simulink model "MotorCtrl_DTC_Math"  (R2023b)
settings: Solver=FixedStepDiscrete  StartTime=0.0  StopTime=5  FixedStep=MC_Sim_BaseStep  RelTol=1e-3  EnableMultiTasking=on
values from neighbouring files (symbols this model uses):
  MC_ADC_BitNum = 0.0    [MotorControlDataDictionary_Math.sldd]
  MC_ADC_Offset = 0.0    [MotorControlDataDictionary_Math.sldd]
  MC_ADC_VRef = 1.0    [MotorControlDataDictionary_Math.sldd]
  MC_Const_DutyL = 0.2    [MotorControlDataDictionary_Math.sldd]
  MC_Const_DutyS = 0.8    [MotorControlDataDictionary_Math.sldd]
  MC_CSA_Gain = 1.0    [MotorControlDataDictionary_Math.sldd]
  MC_Input_Vdc = 13.5    [MotorControlDataDictionary_Math.sldd]
  MC_MOS_DeadTime = 1.0E-6    [MotorControlDataDictionary_Math.sldd]
  MC_Motor_Mechinal_Damp = 1.0E-5    [MotorControlDataDictionary_Math.sldd]
  MC_Motor_Mechinal_Fric = 0.0    [MotorControlDataDictionary_Math.sldd]
  MC_Motor_Mechinal_Inertia = 0.0103    [MotorControlDataDictionary_Math.sldd]
  MC_Motor_Phi = 0.0059190254913385806    [MotorControlDataDictionary_Math.sldd]
  MC_Motor_Rotor_Pn = 4.0    [MotorControlDataDictionary_Math.sldd]
  MC_Motor_Stator_Ld = 5.6345E-5    [MotorControlDataDictionary_Math.sldd]
  MC_Motor_Stator_Lq = 5.6345E-5    [MotorControlDataDictionary_Math.sldd]
  MC_Motor_Stator_Rs = 0.0286    [MotorControlDataDictionary_Math.sldd]
  MC_Param_CurrentPI_Ki = 0.0071879639914134473    [MotorControlDataDictionary_Math.sldd]
  MC_Param_CurrentPI_Kp = 0.283220860906427    [MotorControlDataDictionary_Math.sldd]
  MC_Param_CurrentPI_UdInteMax = 7.794228634059948    [MotorControlDataDictionary_Math.sldd]
  MC_Param_CurrentPI_UdInteMin = -7.794228634059948    [MotorControlDataDictionary_Math.sldd]
  MC_Param_CurrentPI_UdMax = 7.794228634059948    [MotorControlDataDictionary_Math.sldd]
  MC_Param_CurrentPI_UdMin = -7.794228634059948    [MotorControlDataDictionary_Math.sldd]
  MC_Param_CurrentPI_UqInteMax = 7.794228634059948    [MotorControlDataDictionary_Math.sldd]
  MC_Param_CurrentPI_UqInteMin = -7.794228634059948    [MotorControlDataDictionary_Math.sldd]
  MC_Param_CurrentPI_UqMax = 7.794228634059948    [MotorControlDataDictionary_Math.sldd]
  MC_Param_CurrentPI_UqMin = -7.794228634059948    [MotorControlDataDictionary_Math.sldd]
  MC_Param_Flux_Gamma = 750000.0    [MotorControlDataDictionary_Math.sldd]
  MC_Param_Flux_Lalpha = 5.6345E-5    [MotorControlDataDictionary_Math.sldd]
  MC_Param_Flux_Lbeta = 5.6345E-5    [MotorControlDataDictionary_Math.sldd]
  MC_Param_Flux_Ralpha = 0.0286    [MotorControlDataDictionary_Math.sldd]
  MC_Param_Flux_Rbeta = 0.0286    [MotorControlDataDictionary_Math.sldd]
  MC_Param_Luen_BEMFalpha = -17747.803709290976    [MotorControlDataDictionary_Math.sldd]
  MC_Param_Luen_BEMFbeta = -17747.803709290976    [MotorControlDataDictionary_Math.sldd]
  MC_Param_Luen_BEMFErr = -8.0    [MotorControlDataDictionary_Math.sldd]
  MC_Param_Luen_Currentalpha = -507.58718608572195    [MotorControlDataDictionary_Math.sldd]
  MC_Param_Luen_Currentbeta = -507.58718608572195    [MotorControlDataDictionary_Math.sldd]
  MC_Param_Luen_CurrentErr = -8.0    [MotorControlDataDictionary_Math.sldd]
  MC_Param_Luen_PLL_Ki = 2.3480975196640594    [MotorControlDataDictionary_Math.sldd]
  MC_Param_Luen_PLL_Kp = 153.24842212633141    [MotorControlDataDictionary_Math.sldd]
  MC_Param_Luen_Voltagealpha = 17747.803709290976    [MotorControlDataDictionary_Math.sldd]
  MC_Param_Luen_Voltagebeta = 17747.803709290976    [MotorControlDataDictionary_Math.sldd]
  MC_Param_PhasetoReal = 500.0    [MotorControlDataDictionary_Math.sldd]
  MC_Param_SMO_CoffA = 0.97462064069571386    [MotorControlDataDictionary_Math.sldd]
  MC_Param_SMO_CoffB = 0.88739018546454884    [MotorControlDataDictionary_Math.sldd]
  MC_Param_SpeedCtrl_IdMax = 60.0    [MotorControlDataDictionary_Math.sldd]
  MC_Param_SpeedCtrl_IdMin = -60.0    [MotorControlDataDictionary_Math.sldd]
  MC_Param_SpeedCtrl_IqMax = 60.0    [MotorControlDataDictionary_Math.sldd]
  MC_Param_SpeedCtrl_IqMin = -60.0    [MotorControlDataDictionary_Math.sldd]
  MC_Param_SpeedPI_Ki = 0.57248683633241571    [MotorControlDataDictionary_Math.sldd]
  MC_Param_SpeedPI_Kp = 9.1114109857344836    [MotorControlDataDictionary_Math.sldd]
  MC_Param_SpeedtoTheta = 5.0E-5    [MotorControlDataDictionary_Math.sldd]
  MC_Param_SVPWM_DutyMax = 0.98    [MotorControlDataDictionary_Math.sldd]
  MC_Param_SVPWM_DutyMin = 0.02    [MotorControlDataDictionary_Math.sldd]
  MC_Param_SVPWM_SampleOffset1 = 0.02    [MotorControlDataDictionary_Math.sldd]
  MC_Param_SVPWM_SampleOffset2 = 0.015    [MotorControlDataDictionary_Math.sldd]
  MC_Param_SVPWM_SampleValid = 0.011999999999999999    [MotorControlDataDictionary_Math.sldd]
  MC_Sample_CurrentNoise = 1.0E-15    [MotorControlDataDictionary_Math.sldd]
  MC_Sample_Rs = 0.002    [MotorControlDataDictionary_Math.sldd]
  MC_Sample_VbusNoise = 1.0E-15    [MotorControlDataDictionary_Math.sldd]
  MC_Sim_BaseStep = 5.0E-8    [MotorControlDataDictionary_Math.sldd]
  MC_Sim_HFTStep = 5.0E-5    [MotorControlDataDictionary_Math.sldd]
  MC_Sim_MFTStep = 0.002    [MotorControlDataDictionary_Math.sldd]
libraries: simulink x29, spsVoltageMeasurementLib x2, spsDCVoltageSourceLib x1, spsGroundLib x1, spsPermanentMagnetSynchronousMachineLib x1, spsSeriesRLCBranchLib x1, spsThreePhaseVIMeasurementLib x1, spsUniversalBridgeLib x1, sps_lib x1
(part 4 of 5)

== system MotorCtrl_DTC_Math/HFTask/smo/getSpeedandTheta ==
  note: 日志：
      | 2025.03.19：反电势正负号识别错误，改正后可以使用
  Ealpha : Inport
  Ebeta : Inport  Port=2
  Add : Sum
  Add1 : Sum
  Add2 : Sum
  Constant : Constant  Value=2*pi  OutDataTypeStr=single
  Delay One Step : Delay  DelayLength=1
  Delay One Step2 : Delay  DelayLength=1
  Gain : Gain  Gain=-1
  Gain1 : Gain  Gain=2*sqrt(2)/2*100
  Gain2 : Gain  Gain=100^2*MC_Sim_HFTStep
  Gain3 : Gain  Gain=MC_Param_SpeedtoTheta
  Gain5 : Gain  Gain=30/(pi*MC_Motor_Rotor_Pn)  OutDataTypeStr=single  RndMeth=Simplest
  Mod : Math  Operator=mod
  Product : Product
  Product1 : Product
  Sin : Trigonometry  OutputSignalType=real
  Sin1 : Trigonometry  Operator=cos  OutputSignalType=real
  Subtract : Sum  Inputs=+-
  Speed : Outport
  Theta : Outport  Port=2
  wires:
  Sin1/1 -> Product/2
  Sin/1 -> Product1/2
  Gain2/1 -> Add/1
  Add/1 -> Delay One Step/1, Add1/2
  Delay One Step/1 -> Add/2
  Gain1/1 -> Add1/1
  Subtract/1 -> Gain2/1, Gain1/1  "SMOErr"
  Gain3/1 -> Add2/1
  Add2/1 -> Mod/1
  Constant/1 -> Mod/2
  Delay One Step2/1 -> Add2/2, [Theta_Last]
  Mod/1 -> Theta/1, Delay One Step2/1  "ThetaSMO"
  Add1/1 -> Gain5/1, Gain3/1  "SpeedSmo"
  [Theta_Last] -> Sin1/1, Sin/1
  Gain/1 -> Product1/1
  Ebeta/1 -> Gain/1
  Ealpha/1 -> Product/1
  Product/1 -> Subtract/1  "SMOSin"
  Product1/1 -> Subtract/2  "SMOCos"
  Gain5/1 -> Speed/1  "SpeedSMO_RPM"

== system MotorCtrl_DTC_Math/HFTask/svpwm/getVoltageExchange ==
  Valpha : Inport
  Vbeta : Inport  Port=2
  Vdc : Inport  Port=3
  Add : Sum
  Add1 : Sum
  Divide : Product  Inputs=*/
  Divide1 : Product  Inputs=*/
  Gain : Gain  Gain=-1/2
  Gain1 : Gain  Gain=sqrt(3)/2
  Gain2 : Gain  Gain=-1
  Relational Operator : RelationalOperator  OutDataTypeStr=boolean  RndMeth=Simplest  InputSameDT=off
  Relational Operator1 : RelationalOperator  OutDataTypeStr=boolean  RndMeth=Simplest  InputSameDT=off
  Relational Operator2 : RelationalOperator  Operator=<=  OutDataTypeStr=boolean  RndMeth=Simplest  InputSameDT=off
  Relational Operator3 : RelationalOperator  Operator=<=  OutDataTypeStr=boolean  RndMeth=Simplest  InputSameDT=off
  Signal Copy : SignalConversion  OverrideOpt=off
  Subtract : Sum  Inputs=+-
  Switch{,1..3} (4 alike) : Switch  Criteria=u2 > Threshold  SaturateOnIntegerOverflow=off  InputSameDT=off
  getSectorN : Subsystem  Commented=on
  Va : Outport
  Vb : Outport  Port=2
  Vc : Outport  Port=3
  Vmed : Outport  Port=4
  wires:
  Valpha/1 -> Divide/1
  Vbeta/1 -> Divide1/1
  Vdc/1 -> Divide/2, Divide1/2
  Subtract/1 -> Relational Operator3/2, Switch3/3, Relational Operator1/2, Switch1/3, Vc/1  "Vc"
  Add/1 -> Switch2/3, Relational Operator2/2, Switch/3, Relational Operator/2, Vb/1  "Vb"
  Gain1/1 -> Subtract/2, Add/2
  Gain/1 -> Add/1, Subtract/1
  Divide1/1 -> Gain1/1
  Divide/1 -> Gain/1, Signal Copy/1
  Signal Copy/1 -> Switch2/1, Relational Operator2/1, Switch/1, Relational Operator/1, Va/1  "Va"
  Switch1/1 -> Add1/1  "Vmax"
  Relational Operator1/1 -> Switch1/2
  Switch/1 -> Relational Operator1/1, Switch1/1
  Relational Operator/1 -> Switch/2
  Switch3/1 -> Add1/2  "Vmin"
  Relational Operator3/1 -> Switch3/2
  Switch2/1 -> Switch3/1, Relational Operator3/1
  Relational Operator2/1 -> Switch2/2
  Add1/1 -> Gain2/1
  Gain2/1 -> Vmed/1  "Vmed"

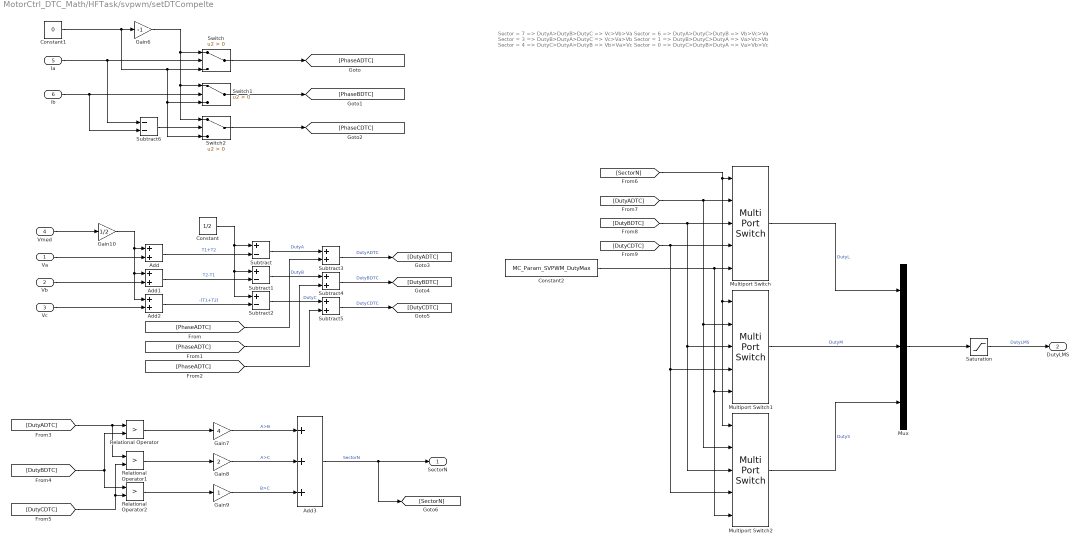
== system MotorCtrl_DTC_Math/HFTask/svpwm/setDTCompelte ==
  note: Sector = 7 => DutyA>DutyB>DutyC => Vc>Vb>Va
      | Sector = 6 => DutyA>DutyC>DutyB => Vb>Vc>Va
      | Sector = 3 => DutyB>DutyA>DutyC => Vc>Va>Vb
      | Sector = 1 => DutyB>DutyC>DutyA => Va>Vc>Vb
      | Sector = 4 => DutyC>DutyA>DutyB => Vb>Va>Vc
      | Sector = 0 => DutyC>DutyB>DutyA => Va>Vb>Vc
  Va : Inport
  Vb : Inport  Port=2
  Vc : Inport  Port=3
  Vmed : Inport  Port=4
  Ia : Inport  Port=5
  ib : Inport  Port=6
  Add : Sum
  Add1 : Sum
  Add2 : Sum
  Add3 : Sum  Inputs=+++
  Constant : Constant  Value=1/2  OutDataTypeStr=single  SampleTime=MC_Sim_HFTStep
  Constant1 : Constant  Value=0  OutDataTypeStr=single
  Constant2 : Constant  Value=MC_Param_SVPWM_DutyMax  OutDataTypeStr=single
  Gain10 : Gain  Gain=1/2
  Gain6 : Gain  Gain=-1
  Gain7 : Gain  Gain=4  OutDataTypeStr=single  RndMeth=Simplest
  Gain8 : Gain  Gain=2  OutDataTypeStr=single  RndMeth=Simplest
  Gain9 : Gain  OutDataTypeStr=single  RndMeth=Simplest
  Multiport Switch : MultiPortSwitch  DataPortOrder=Specify indices  DataPortIndices={[6,7],[1,3],[0,4]}  DataPortForDefault=Additional data port  SaturateOnIntegerOverflow=off  InputSameDT=off
  Multiport Switch1 : MultiPortSwitch  DataPortOrder=Specify indices  DataPortIndices={[4,3],[7,0],[6,1]}  DataPortForDefault=Additional data port  SaturateOnIntegerOverflow=off  InputSameDT=off
  Multiport Switch2 : MultiPortSwitch  DataPortOrder=Specify indices  DataPortIndices={[0,1],[4,6],[3,7]}  DataPortForDefault=Additional data port  SaturateOnIntegerOverflow=off  InputSameDT=off
  Mux : Mux  Inputs=3
  Relational Operator : RelationalOperator  Operator=>  OutDataTypeStr=boolean  RndMeth=Simplest  InputSameDT=off
  Relational Operator1 : RelationalOperator  Operator=>  OutDataTypeStr=boolean  RndMeth=Simplest  InputSameDT=off
  Relational Operator2 : RelationalOperator  Operator=>  OutDataTypeStr=boolean  RndMeth=Simplest  InputSameDT=off
  Saturation : Saturate  UpperLimit=MC_Param_SVPWM_DutyMax-(MC_MOS_DeadTime/MC_Sim_HFTStep)  LowerLimit=MC_Param_SVPWM_DutyMin+(MC_MOS_DeadTime/MC_Sim_HFTStep)
      settings: AttributesFormatString=|
      | OutputMax = %<UpperLimit>
      | OutputMin = %<LowerLimit>
  Subtract : Sum  Inputs=+-
  Subtract1 : Sum  Inputs=+-
  Subtract2 : Sum  Inputs=+-
  Subtract3 : Sum
  Subtract4 : Sum
  Subtract5 : Sum
  Subtract6 : Sum  Inputs=--
  Switch : Switch  Criteria=u2 > Threshold  SaturateOnIntegerOverflow=off  InputSameDT=off
  Switch1 : Switch  Criteria=u2 > Threshold  SaturateOnIntegerOverflow=off  InputSameDT=off
  Switch2 : Switch  Criteria=u2 > Threshold  SaturateOnIntegerOverflow=off  InputSameDT=off
  SectorN : Outport
  DutyLMS : Outport  Port=2
  wires:
  Va/1 -> Add/2
  Vmed/1 -> Gain10/1
  Vb/1 -> Add1/2
  Vc/1 -> Add2/2
  Add/1 -> Subtract/2  "T1+T2"
  Add2/1 -> Subtract2/2  "-(T1+T2)"
  Add1/1 -> Subtract1/2  "T2-T1"
  Constant/1 -> Subtract2/1, Subtract1/1, Subtract/1
  Subtract/1 -> Subtract3/1  "DutyA"
  Subtract1/1 -> Subtract4/1  "DutyB"
  Subtract2/1 -> Subtract5/1  "DutyC"
  Ia/1 -> Subtract6/1, Switch/2
  Gain6/1 -> Switch2/1, Switch1/1, Switch/1
  ib/1 -> Subtract6/2, Switch1/2
  Subtract6/1 -> Switch2/2
  Constant1/1 -> Switch2/3, Switch1/3, Switch/3, Gain6/1
  Switch/1 -> [PhaseADTC]
  Switch1/1 -> [PhaseBDTC]
  Switch2/1 -> [PhaseCDTC]
  [PhaseADTC] -> Subtract3/2
  [PhaseADTC] -> Subtract4/2
  [PhaseADTC] -> Subtract5/2
  [DutyBDTC] -> Relational Operator/2, Relational Operator2/1
  [DutyADTC] -> Relational Operator1/1, Relational Operator/1
  [DutyCDTC] -> Relational Operator2/2, Relational Operator1/2
  Relational Operator/1 -> Gain7/1
  Relational Operator1/1 -> Gain8/1
  Relational Operator2/1 -> Gain9/1
  Gain8/1 -> Add3/2  "A>C"
  Gain9/1 -> Add3/3  "B>C"
  Gain7/1 -> Add3/1  "A>B"
  Add3/1 -> [SectorN], SectorN/1  "SectorN"
  Gain10/1 -> Add2/1, Add1/1, Add/1
  Subtract3/1 -> [DutyADTC]  "DutyADTC"
  Subtract4/1 -> [DutyBDTC]  "DutyBDTC"
  Subtract5/1 -> [DutyCDTC]  "DutyCDTC"
  [SectorN] -> Multiport Switch2/1, Multiport Switch1/1, Multiport Switch/1
  Multiport Switch/1 -> Mux/1  "DutyL"
  Constant2/1 -> Multiport Switch2/5, Multiport Switch1/5, Multiport Switch/5
  Multiport Switch1/1 -> Mux/2  "DutyM"
  Multiport Switch2/1 -> Mux/3  "DutyS"
  Mux/1 -> Saturation/1
  Saturation/1 -> DutyLMS/1  "DutyLMS"
  [DutyADTC] -> Multiport Switch2/2, Multiport Switch1/2, Multiport Switch/2
  [DutyCDTC] -> Multiport Switch2/4, Multiport Switch1/4, Multiport Switch/4
  [DutyBDTC] -> Multiport Switch2/3, Multiport Switch1/3, Multiport Switch/3

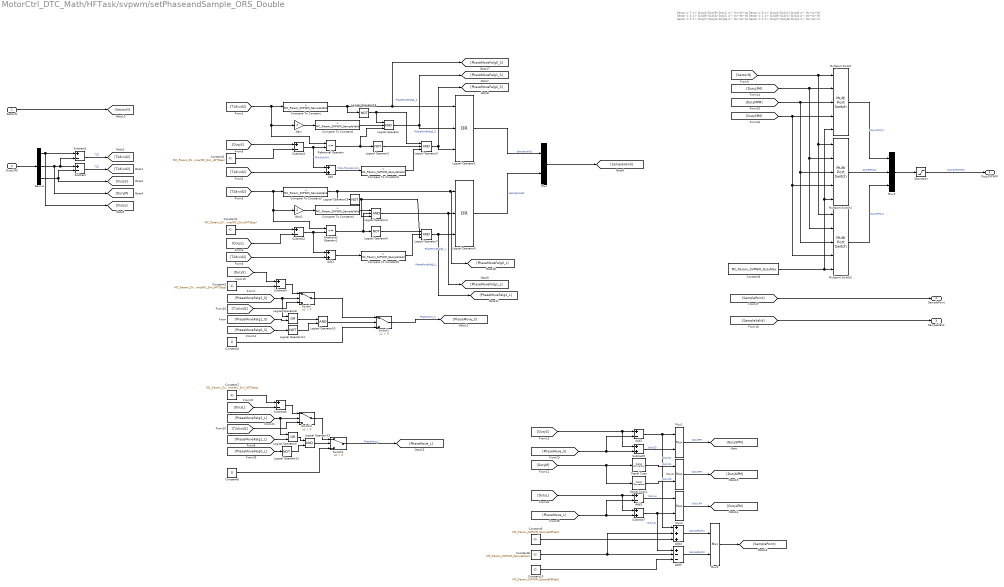
== system MotorCtrl_DTC_Math/HFTask/svpwm/setPhaseandSample_ORS_Double ==
  note: Sector = 7 => DutyA>DutyB>DutyC => Vc>Vb>Va
      | Sector = 6 => DutyA>DutyC>DutyB => Vb>Vc>Va
      | Sector = 3 => DutyB>DutyA>DutyC => Vc>Va>Vb
      | Sector = 1 => DutyB>DutyC>DutyA => Va>Vc>Vb
      | Sector = 4 => DutyC>DutyA>DutyB => Vb>Va>Vc
      | Sector = 0 => DutyC>DutyB>DutyA => Va>Vb>Vc
  SectorN : Inport
  DutyLMS : Inport  Port=2
  Add : Sum
  Add1 : Sum
  Add2 : Sum  Inputs=+-
  Add3 : Sum  Inputs=+-
  Add4 : Sum  Inputs=+++
  Add5 : Sum  Inputs=+--
  Compare To Constant{,1..5} (6 alike) : simulink/Logic and Bit Operations/Compare To Constant  relop=>  const=MC_Param_SVPWM_SampleValid  OutDataTypeStr=boolean
  Constant1 : Constant  Value=MC_Param_SVPWM_DutyMax-(MC_MOS_DeadTime/MC_Sim_HFTStep)  OutDataTypeStr=single
  Constant10 : Constant  Value=MC_Param_SVPWM_SampleOffset2  OutDataTypeStr=single
  Constant2 : Constant  Value=MC_Param_SVPWM_DutyMin+(MC_MOS_DeadTime/MC_Sim_HFTStep)  OutDataTypeStr=single
  Constant3 : Constant  Value=MC_Param_SVPWM_DutyMin+(MC_MOS_DeadTime/MC_Sim_HFTStep)  OutDataTypeStr=single
  Constant4 : Constant  Value=0  OutDataTypeStr=single
  Constant5 : Constant  Value=MC_Param_SVPWM_DutyMax  OutDataTypeStr=single
  Constant6 : Constant  Value=0  OutDataTypeStr=single
  Constant7 : Constant  Value=MC_Param_SVPWM_DutyMax-(MC_MOS_DeadTime/MC_Sim_HFTStep)  OutDataTypeStr=single
  Constant8 : Constant  Value=MC_Param_SVPWM_SampleValid  OutDataTypeStr=single
  Constant9 : Constant  Value=MC_Param_SVPWM_SampleOffset1  OutDataTypeStr=single
  Demux : Demux  Outputs=3
  Gain : Gain  Gain=2
  Gain1 : Gain  Gain=2
  Logical Operator{,3..4,7} (4 alike) : Logic  Inputs=3  AllPortsSameDT=off  OutDataTypeStr=boolean
  Logical Operator1 : Logic  Operator=OR  Inputs=3  AllPortsSameDT=off  OutDataTypeStr=boolean
  Logical Operator10 : Logic  AllPortsSameDT=off  OutDataTypeStr=boolean
  Logical Operator{2,6,11..12,14..15} (6 alike) : Logic  Operator=NOT  AllPortsSameDT=off  OutDataTypeStr=boolean
  Logical Operator13 : Logic  AllPortsSameDT=off  OutDataTypeStr=boolean
  Logical Operator5 : Logic  Operator=OR  Inputs=3  AllPortsSameDT=off  OutDataTypeStr=boolean
  Logical Operator8 : Logic  Operator=OR  AllPortsSameDT=off  OutDataTypeStr=boolean
  Logical Operator9 : Logic  Operator=OR  AllPortsSameDT=off  OutDataTypeStr=boolean
  Multiport Switch : MultiPortSwitch  DataPortOrder=Specify indices  DataPortIndices={[7,6],[3,4],[0,1]}  DataPortForDefault=Additional data port  SaturateOnIntegerOverflow=off  InputSameDT=off
  Multiport Switch1 : MultiPortSwitch  DataPortOrder=Specify indices  DataPortIndices={[3,1],[7,0],[6,4]}  DataPortForDefault=Additional data port  SaturateOnIntegerOverflow=off  InputSameDT=off
  Multiport Switch2 : MultiPortSwitch  DataPortOrder=Specify indices  DataPortIndices={[4,0],[6,1],[7,3]}  DataPortForDefault=Additional data port  SaturateOnIntegerOverflow=off  InputSameDT=off
  Mux{,1..4} (5 alike) : Mux  Inputs=2
  Mux5 : Mux  Inputs=3
  Relational Operator : RelationalOperator  Operator=<=  OutDataTypeStr=boolean  RndMeth=Simplest  InputSameDT=off
  Relational Operator1 : RelationalOperator  Operator=<=  OutDataTypeStr=boolean  RndMeth=Simplest  InputSameDT=off
  Saturation : Saturate  UpperLimit=MC_Param_SVPWM_DutyMax  LowerLimit=MC_Param_SVPWM_DutyMin
      settings: AttributesFormatString=|
      | OutputMax = %<UpperLimit>
      | OutputMin = %<LowerLimit>
  Signal Copy : SignalConversion  OverrideOpt=off
  Signal Copy1 : SignalConversion  OverrideOpt=off
  Subtract{,1..4,6} (6 alike) : Sum  Inputs=+-
  Subtract5 : Sum
  Subtract7 : Sum
  Switch{,1..3} (4 alike) : Switch  Criteria=u2 > Threshold  SaturateOnIntegerOverflow=off  InputSameDT=off
  DutySVPWM : Outport
  SamplePoint : Outport  Port=2
  SampleValid : Outport  Port=3
  wires:
  DutyLMS/1 -> Demux/1
  Subtract/1 -> [T1divid2]  "T1/2"
  Subtract1/1 -> [T2divid2]  "T2/2"
  SectorN/1 -> [SectorN]
  [SectorN] -> Multiport Switch2/1, Multiport Switch1/1, Multiport Switch/1
  [DutyLPM] -> Multiport Switch2/2, Multiport Switch1/2, Multiport Switch/2
  [DutyMPM] -> Multiport Switch2/3, Multiport Switch1/3, Multiport Switch/3
  [DutySPM] -> Multiport Switch1/4, Multiport Switch2/4, Multiport Switch/4
  Constant5/1 -> Multiport Switch1/5, Multiport Switch/5, Multiport Switch2/5
  Multiport Switch1/1 -> Mux5/2  "DutyBPM[2]"
  Multiport Switch2/1 -> Mux5/3  "DutyCPM[2]"
  Multiport Switch/1 -> Mux5/1  "DutyAPM[2]"
  [SamplePoint] -> SamplePoint/1
  [SampleValid] -> SampleValid/1
  Mux5/1 -> Saturation/1
  Saturation/1 -> DutySVPWM/1  "DutySVPWM[6]"
  [T1divid2] -> Relational Operator/1, Gain/1, Compare To Constant/1
  Gain/1 -> Compare To Constant1/1
  [DutyS] -> Subtract3/1
  Subtract3/1 -> Add/1, Relational Operator/2  "T0/4-DutyMin"
  Relational Operator/1 -> Logical Operator/3, Logical Operator2/1
  Logical Operator/1 -> Logical Operator1/2, [PhaseMoveFalg1_S]  "PhaseMoveFalg1_S"
  [T1divid2] -> Add/2
  Add/1 -> Compare To Constant2/1  "T1/2+T0/4-DutyMin"
  Compare To Constant/1 -> Logical Operator14/1, [PhaseMoveFalg0_S], Logical Operator1/1
  Logical Operator1/1 -> Mux/1  "SampleValid1"
  Logical Operator5/1 -> Mux/2  "SampleValid2"
  Compare To Constant3/1 -> Logical Operator15/1, [PhaseMoveFalg0_L], Logical Operator5/1
  Compare To Constant5/1 -> Logical Operator7/2
  Logical Operator6/1 -> Logical Operator7/1
  Logical Operator7/1 -> [PhaseMoveFalg2_L], Logical Operator5/3  "PhaseMoveFalg2_L"
  Add1/1 -> Compare To Constant5/1
  [T2divid2] -> Add1/2
  Logical Operator4/1 -> [PhaseMoveFalg1_L], Logical Operator5/2  "PhaseMoveFalg1_L"
  Relational Operator1/1 -> Logical Operator4/2, Logical Operator6/1
  Compare To Constant4/1 -> Logical Operator4/1
  Subtract2/1 -> Relational Operator1/2, Add1/1
  Constant1/1 -> Subtract2/1
  [DutyL] -> Subtract2/2
  Gain1/1 -> Compare To Constant4/1
  [T2divid2] -> Compare To Constant3/1, Gain1/1, Relational Operator1/1
  Constant2/1 -> Subtract3/2
  Mux/1 -> [SampleValid]
  Logical Operator3/1 -> Logical Operator1/3, [PhaseMoveFalg2_S]  "PhaseMoveFalg2_S"
  Constant3/1 -> Subtract4/2
  [DutyS] -> Subtract4/1
  [PhaseMoveFalg2_S] -> Logical Operator8/1, Switch/2
  Switch/1 -> Switch1/1
  Constant4/1 -> Switch1/3
  Switch1/1 -> [PhaseMove_S]  "PhaseMove_S"
  [T1divid2] -> Switch/3
  Subtract4/1 -> Switch/1
  Switch2/1 -> [PhaseMove_L]  "PhaseMove_L"
  Constant6/1 -> Switch2/3
  [T2divid2] -> Switch3/3
  Switch3/1 -> Switch2/1
  [DutyL] -> Subtract6/2
  Constant7/1 -> Subtract6/1
  Subtract6/1 -> Switch3/1
  Demux/1 -> [DutyL], Subtract1/1
  Demux/2 -> [DutyM], Subtract1/2, Subtract/1
  Demux/3 -> Subtract/2, [DutyS]
  [DutyS] -> Subtract5/1, Add2/1
  [PhaseMove_S] -> Add2/2, Subtract5/2
  Add2/1 -> Mux1/1, Add4/1  "DutySU"
  Subtract5/1 -> Mux1/2  "DutySD"
  Subtract7/1 -> Add5/1, Mux2/2  "DutyLD"
  Add3/1 -> Mux2/1  "DutyLU"
  [PhaseMove_L] -> Subtract7/2, Add3/2
  [DutyL] -> Add3/1, Subtract7/1
  [DutyM] -> Signal Copy1/1, Signal Copy/1
  Signal Copy1/1 -> Mux3/2  "DutyMD"
  Signal Copy/1 -> Mux3/1  "DutyMU"
  Mux1/1 -> [DutySPM]  "DutySPM"
  Mux2/1 -> [DutyLPM]  "DutyLPM"
  Mux3/1 -> [DutyMPM]  "DutyMPM"
  Constant8/1 -> Add4/2, Add5/2
  Add4/1 -> Mux4/1  "SamplePoint1"
  Add5/1 -> Mux4/2  "SamplePoint2"
  Mux4/1 -> [SamplePoint]
  Constant9/1 -> Add4/3
  Constant10/1 -> Add5/3
  [PhaseMoveFalg2_L] -> Logical Operator9/1, Switch3/2
  [PhaseMoveFalg1_L] -> Logical Operator9/2
  Logical Operator10/1 -> Switch1/2
  Logical Operator8/1 -> Logical Operator10/1
  [PhaseMoveFalg0_S] -> Logical Operator11/1
  Logical Operator11/1 -> Logical Operator10/2
  [PhaseMoveFalg1_S] -> Logical Operator8/2
  [PhaseMoveFalg0_L] -> Logical Operator12/1
  Logical Operator13/1 -> Switch2/2
  Logical Operator9/1 -> Logical Operator13/1
  Logical Operator12/1 -> Logical Operator13/2
  Compare To Constant1/1 -> Logical Operator/2
  Logical Operator14/1 -> Logical Operator3/1, Logical Operator/1
  Logical Operator2/1 -> Logical Operator3/2
  Compare To Constant2/1 -> Logical Operator3/3
  Logical Operator15/1 -> Logical Operator4/3, Logical Operator7/3

== system MotorCtrl_DTC_Math/Hardware_Math/PWMGenerate/DeadTimeGenerate ==
  FLag : Inport
  DutyABC : Inport  Port=2
  APhaseDeadTime : Subsystem
  BPhaseDeadTime : Subsystem
  CPhaseDeadTime : Subsystem
  Constant : Constant  Value=MC_MOS_DeadTime/MC_Sim_HFTStep  SampleTime=-1
  Demux : Demux  Outputs=6
  GateAH : Outport
  GateAL : Outport  Port=2
  GateBH : Outport  Port=3
  GateBL : Outport  Port=4
  GateCH : Outport  Port=5
  GateCL : Outport  Port=6
  wires:
  Demux/6 -> CPhaseDeadTime/3(CL)
  DutyABC/1 -> Demux/1
  CPhaseDeadTime/1(CDH) -> GateCH/1
  CPhaseDeadTime/2(CDL) -> GateCL/1
  BPhaseDeadTime/1(BDH) -> GateBH/1
  BPhaseDeadTime/2(BDL) -> GateBL/1
  APhaseDeadTime/2(ADL) -> GateAL/1
  FLag/1 -> CPhaseDeadTime/1(FLag), BPhaseDeadTime/1(FLag), APhaseDeadTime/1(FLag)
  Constant/1 -> APhaseDeadTime/4(DeadTime), BPhaseDeadTime/4(DeadTime), CPhaseDeadTime/4(DeadTime)
  APhaseDeadTime/1(ADH) -> GateAH/1
  Demux/5 -> BPhaseDeadTime/3(BL)
  Demux/4 -> APhaseDeadTime/3(AL)
  Demux/1 -> APhaseDeadTime/2(AH)
  Demux/2 -> BPhaseDeadTime/2(BH)
  Demux/3 -> CPhaseDeadTime/2(CH)

== system MotorCtrl_DTC_Math/Hardware_Math/currentSample/getCurrentSample_ORS_Double ==
  SampleTrigger : Inport
  Current : Inport  Port=2
  Demux : Demux  Outputs=2
  Mux : Mux  Inputs=2
  getCurrentSample1 : Subsystem  TreatAsAtomicUnit=on
  getCurrentSample2 : Subsystem  TreatAsAtomicUnit=on
  SampleCurrent : Outport
  wires:
  SampleTrigger/1 -> Demux/1
  Demux/1 -> getCurrentSample1/Trigger
  Demux/2 -> getCurrentSample2/Trigger
  Current/1 -> getCurrentSample2/1(Current), getCurrentSample1/1(Current)
  getCurrentSample1/1(SampleCurrentUp) -> Mux/1
  Mux/1 -> SampleCurrent/1
  getCurrentSample2/1(SampleCurrentDown) -> Mux/2

== system MotorCtrl_DTC_Math/Hardware_Math/currentSample/getCurrentSample_ORS_Single ==
  SampleTrigger : Inport
  Current : Inport  Port=2
  Demux : Demux  Outputs=2
  Mux : Mux  Inputs=2
  getCurrentSample1 : Subsystem  TreatAsAtomicUnit=on
  getCurrentSample2 : Subsystem  TreatAsAtomicUnit=on
  SampleCurrent : Outport
  wires:
  SampleTrigger/1 -> Demux/1
  Mux/1 -> SampleCurrent/1
  getCurrentSample1/1(SampleCurrentUp) -> Mux/1
  getCurrentSample2/1(SampleCurrentDown) -> Mux/2
  Demux/1 -> getCurrentSample1/Trigger
  Demux/2 -> getCurrentSample2/Trigger
  Current/1 -> getCurrentSample2/1(Current), getCurrentSample1/1(Current)

== system MotorCtrl_DTC_Math/Hardware_Math/currentSample/getCurrentSample_TRS(Three) ==
  SampleTrigger : Inport
  Current : Inport  Port=2
  Demux : Demux  Outputs=3
  Mux : Mux  Inputs=3
  getCurrentSampleA : Subsystem  TreatAsAtomicUnit=on
  getCurrentSampleB : Subsystem  TreatAsAtomicUnit=on
  getCurrentSampleC : Subsystem  TreatAsAtomicUnit=on
  SampleCurrent : Outport
  wires:
  getCurrentSampleA/1(SampleCurrentA) -> Mux/1
  getCurrentSampleB/1(SampleCurrentB) -> Mux/2
  Mux/1 -> SampleCurrent/1
  getCurrentSampleC/1(SampleCurrentC) -> Mux/3
  SampleTrigger/1 -> getCurrentSampleB/Trigger, getCurrentSampleC/Trigger, getCurrentSampleA/Trigger
  Current/1 -> Demux/1
  Demux/1 -> getCurrentSampleA/1(Current)
  Demux/2 -> getCurrentSampleB/1(Current)
  Demux/3 -> getCurrentSampleC/1(Current)

== system MotorCtrl_DTC_Math/Hardware_Math/currentSample/getCurrentSample_TRS(Two) ==
  SampleTrigger : Inport
  Current : Inport  Port=2
  Demux : Demux  Outputs=2
  Mux : Mux  Inputs=2
  getCurrentSample1 : Subsystem  TreatAsAtomicUnit=on
  getCurrentSample2 : Subsystem  TreatAsAtomicUnit=on
  SampleCurrent : Outport
  wires:
  Demux/1 -> getCurrentSample1/Trigger
  Current/1 -> getCurrentSample2/1(Current), getCurrentSample1/1(Current)
  Demux/2 -> getCurrentSample2/Trigger
  getCurrentSample1/1(SampleCurrentUp) -> Mux/1
  getCurrentSample2/1(SampleCurrentDown) -> Mux/2
  Mux/1 -> SampleCurrent/1
  SampleTrigger/1 -> Demux/1

== system MotorCtrl_DTC_Math/svpwm_OM/getVoltageExchange/getSectorN ==
  Valpha : Inport
  Vbeta : Inport  Port=2
  Add : Sum
  Add1 : Sum  Inputs=+++
  Constant : Constant
  Constant1 : Constant  Value=0
  Gain : Gain  Gain=sqrt(3)/2
  Gain1 : Gain  Gain=-1/2
  Gain2 : Gain
  Gain3 : Gain  Gain=2
  Gain4 : Gain  Gain=4
  Subtract : Sum  Inputs=-+
  Switch : Switch  Criteria=u2 > Threshold  SaturateOnIntegerOverflow=off  InputSameDT=off
  Switch1 : Switch  Criteria=u2 > Threshold  SaturateOnIntegerOverflow=off  InputSameDT=off
  Switch2 : Switch  Criteria=u2 > Threshold  SaturateOnIntegerOverflow=off  InputSameDT=off
  SectorN : Outport
  wires:
  Add1/1 -> SectorN/1  "SectorN"
  Gain4/1 -> Add1/1
  Add/1 -> Switch1/2  "U2"
  Switch2/1 -> Gain4/1
  Gain2/1 -> Add1/3
  Subtract/1 -> Switch2/2  "U3"
  Valpha/1 -> Gain/1
  Constant1/1 -> Switch/3, Switch1/3, Switch2/3
  Vbeta/1 -> Gain1/1, Switch/2  "U1"
  Switch1/1 -> Gain3/1
  Gain/1 -> Subtract/1, Add/1
  Switch/1 -> Gain2/1
  Gain1/1 -> Subtract/2, Add/2
  Gain3/1 -> Add1/2
  Constant/1 -> Switch2/1, Switch/1, Switch1/1

== system MotorCtrl_DTC_Math/HFTask/svpwm/getVoltageExchange/getSectorN ==
  Valpha : Inport
  Vbeta : Inport  Port=2
  Add : Sum
  Add1 : Sum  Inputs=+++
  Constant : Constant
  Constant1 : Constant  Value=0
  Gain : Gain  Gain=sqrt(3)/2
  Gain1 : Gain  Gain=-1/2
  Gain2 : Gain
  Gain3 : Gain  Gain=2
  Gain4 : Gain  Gain=4
  Subtract : Sum  Inputs=-+
  Switch : Switch  Criteria=u2 > Threshold  SaturateOnIntegerOverflow=off  InputSameDT=off
  Switch1 : Switch  Criteria=u2 > Threshold  SaturateOnIntegerOverflow=off  InputSameDT=off
  Switch2 : Switch  Criteria=u2 > Threshold  SaturateOnIntegerOverflow=off  InputSameDT=off
  SectorN : Outport
  wires:
  Constant/1 -> Switch1/1, Switch/1, Switch2/1
  Gain3/1 -> Add1/2
  Gain1/1 -> Add/2, Subtract/2
  Switch/1 -> Gain2/1
  Gain/1 -> Add/1, Subtract/1
  Switch1/1 -> Gain3/1
  Vbeta/1 -> Switch/2, Gain1/1  "U1"
  Constant1/1 -> Switch2/3, Switch1/3, Switch/3
  Valpha/1 -> Gain/1
  Subtract/1 -> Switch2/2  "U3"
  Gain2/1 -> Add1/3
  Switch2/1 -> Gain4/1
  Add/1 -> Switch1/2  "U2"
  Gain4/1 -> Add1/1
  Add1/1 -> SectorN/1  "SectorN"

== system MotorCtrl_DTC_Math/Hardware_Math/PWMGenerate/DeadTimeGenerate/APhaseDeadTime ==
  FLag : Inport
  AH : Inport  Port=2
  AL : Inport  Port=3
  DeadTime : Inport  Port=4
  Add : Sum
  Subtract : Sum  Inputs=+-
  Switch : Switch  Criteria=u2 > Threshold  SaturateOnIntegerOverflow=off  InputSameDT=off
  Switch1 : Switch  Criteria=u2 > Threshold  SaturateOnIntegerOverflow=off  InputSameDT=off
  ADH : Outport
  ADL : Outport  Port=2
  wires:
  DeadTime/1 -> Add/2, Subtract/2
  AL/1 -> Switch/3, Subtract/1
  FLag/1 -> Switch/2, Switch1/2
  Add/1 -> Switch/1
  Switch/1 -> ADH/1  "ADH"
  AH/1 -> Switch1/1, Add/1
  Subtract/1 -> Switch1/3
  Switch1/1 -> ADL/1  "ADL"

== system MotorCtrl_DTC_Math/Hardware_Math/PWMGenerate/DeadTimeGenerate/BPhaseDeadTime ==
  FLag : Inport
  BH : Inport  Port=2
  BL : Inport  Port=3
  DeadTime : Inport  Port=4
  Add : Sum
  Subtract : Sum  Inputs=+-
  Switch : Switch  Criteria=u2 > Threshold  SaturateOnIntegerOverflow=off  InputSameDT=off
  Switch1 : Switch  Criteria=u2 > Threshold  SaturateOnIntegerOverflow=off  InputSameDT=off
  BDH : Outport
  BDL : Outport  Port=2
  wires:
  Switch1/1 -> BDL/1  "BDL"
  Subtract/1 -> Switch1/3
  BH/1 -> Switch1/1, Add/1
  Switch/1 -> BDH/1  "BDH"
  Add/1 -> Switch/1
  FLag/1 -> Switch1/2, Switch/2
  BL/1 -> Subtract/1, Switch/3
  DeadTime/1 -> Subtract/2, Add/2

== system MotorCtrl_DTC_Math/Hardware_Math/PWMGenerate/DeadTimeGenerate/CPhaseDeadTime ==
  FLag : Inport
  CH : Inport  Port=2
  CL : Inport  Port=3
  DeadTime : Inport  Port=4
  Add : Sum
  Subtract : Sum  Inputs=+-
  Switch : Switch  Criteria=u2 > Threshold  SaturateOnIntegerOverflow=off  InputSameDT=off
  Switch1 : Switch  Criteria=u2 > Threshold  SaturateOnIntegerOverflow=off  InputSameDT=off
  CDH : Outport
  CDL : Outport  Port=2
  wires:
  DeadTime/1 -> Add/2, Subtract/2
  CL/1 -> Switch/3, Subtract/1
  FLag/1 -> Switch/2, Switch1/2
  Add/1 -> Switch/1
  Switch/1 -> CDH/1  "CDH"
  CH/1 -> Switch1/1, Add/1
  Subtract/1 -> Switch1/3
  Switch1/1 -> CDL/1  "CDL"

== system MotorCtrl_DTC_Math/Hardware_Math/currentSample/getCurrentSample_ORS_Double/getCurrentSample1 ==
  Current : Inport
  Trigger : TriggerPort  VariantControl=(inherit)
  ADCOffset : Constant  Value=MC_ADC_Offset  SampleTime=-1
  ADCQuality : Gain  Gain=2^MC_ADC_BitNum/MC_ADC_VRef
  Add : Sum
  CSAGain : Gain  Gain=MC_CSA_Gain
  Data Type Conversion3 : DataTypeConversion  OutDataTypeStr=single  SaturateOnIntegerOverflow=off  RndMeth=Floor
  SampleCurrentUp : Outport
  wires:
  ADCQuality/1 -> Data Type Conversion3/1
  ADCOffset/1 -> Add/1
  Add/1 -> ADCQuality/1
  CSAGain/1 -> Add/2
  Data Type Conversion3/1 -> SampleCurrentUp/1  "SampleCurrentUp"
  Current/1 -> CSAGain/1

== system MotorCtrl_DTC_Math/Hardware_Math/currentSample/getCurrentSample_ORS_Double/getCurrentSample2 ==
  Current : Inport
  Trigger : TriggerPort  TriggerType=falling  VariantControl=(inherit)
  ADCOffset : Constant  Value=MC_ADC_Offset  SampleTime=-1
  ADCQuality : Gain  Gain=2^MC_ADC_BitNum/MC_ADC_VRef
  Add : Sum
  CSAGain : Gain  Gain=MC_CSA_Gain
  Data Type Conversion3 : DataTypeConversion  OutDataTypeStr=single  SaturateOnIntegerOverflow=off  RndMeth=Floor
  SampleCurrentDown : Outport
  wires:
  Current/1 -> CSAGain/1
  Add/1 -> ADCQuality/1
  Data Type Conversion3/1 -> SampleCurrentDown/1  "SampleCurrentUp"
  ADCOffset/1 -> Add/1
  ADCQuality/1 -> Data Type Conversion3/1
  CSAGain/1 -> Add/2

== system MotorCtrl_DTC_Math/Hardware_Math/currentSample/getCurrentSample_ORS_Single/getCurrentSample1 ==
  Current : Inport
  Trigger : TriggerPort  VariantControl=(inherit)
  ADCOffset : Constant  Value=0  SampleTime=-1
  ADCQuality : Gain
  Add : Sum
  CSAGain : Gain
  Data Type Conversion3 : DataTypeConversion  OutDataTypeStr=single  SaturateOnIntegerOverflow=off  RndMeth=Floor
  SampleCurrentUp : Outport
  wires:
  ADCQuality/1 -> Data Type Conversion3/1
  ADCOffset/1 -> Add/1
  Add/1 -> ADCQuality/1
  CSAGain/1 -> Add/2
  Data Type Conversion3/1 -> SampleCurrentUp/1  "SampleCurrentUp"
  Current/1 -> CSAGain/1

== system MotorCtrl_DTC_Math/Hardware_Math/currentSample/getCurrentSample_ORS_Single/getCurrentSample2 ==
  Current : Inport
  Trigger : TriggerPort  VariantControl=(inherit)
  ADCOffset : Constant  Value=0  SampleTime=-1
  ADCQuality : Gain
  Add : Sum
  CSAGain : Gain
  Data Type Conversion3 : DataTypeConversion  OutDataTypeStr=single  SaturateOnIntegerOverflow=off  RndMeth=Floor
  SampleCurrentDown : Outport
  wires:
  Current/1 -> CSAGain/1
  CSAGain/1 -> Add/2
  Add/1 -> ADCQuality/1
  ADCOffset/1 -> Add/1
  ADCQuality/1 -> Data Type Conversion3/1
  Data Type Conversion3/1 -> SampleCurrentDown/1  "SampleCurrentDown"

== system MotorCtrl_DTC_Math/Hardware_Math/currentSample/getCurrentSample_TRS(Three)/getCurrentSampleA ==
  Current : Inport
  Trigger : TriggerPort  TriggerType=falling  VariantControl=(inherit)
  ADCOffset : Constant  Value=0  SampleTime=-1
  ADCQuality : Gain
  Add : Sum
  CSAGain : Gain
  Data Type Conversion3 : DataTypeConversion  OutDataTypeStr=single  SaturateOnIntegerOverflow=off  RndMeth=Floor
  SampleCurrentA : Outport
  wires:
  ADCQuality/1 -> Data Type Conversion3/1
  ADCOffset/1 -> Add/1
  Add/1 -> ADCQuality/1
  CSAGain/1 -> Add/2
  Data Type Conversion3/1 -> SampleCurrentA/1  "SampleCurrentA"
  Current/1 -> CSAGain/1
